simulink model "Lab6CorreguidoMAL"  (R2017b)
settings: Solver=VariableStepAuto  StartTime=0.0  StopTime=10000  RelTol=1e-3
settings Model: Creator=Cx001la  LastModifiedBy=Cx001la

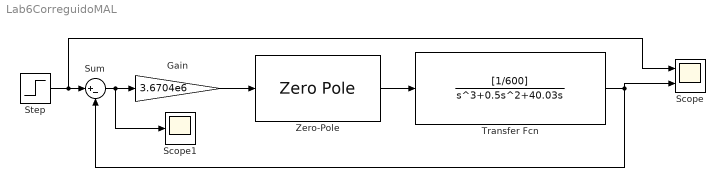
== system Lab6CorreguidoMAL ==
  Gain : Gain  Gain=3.6704e6
  Scope : Scope  NumInputPorts=2
  Scope1 : Scope
  Step : Step  Time=0  SampleTime=0
  Sum : Sum  Inputs=|+-
  Transfer Fcn : TransferFcn  Numerator=[1/600]  Denominator=[1 0.5 40.03 0]
  Zero-Pole : ZeroPole  Zeros=[-2.17 -2.17 -2.17 -2.17 -2.17 ]  Poles=[-18.0788 -18.0788 -18.0788 -18.0788 -18.0788 ]
  wires:
  Step/1 -> Scope/1, Sum/1
  Sum/1 -> Scope1/1, Gain/1
  Gain/1 -> Zero-Pole/1
  Zero-Pole/1 -> Transfer Fcn/1
  Transfer Fcn/1 -> Scope/2, Sum/2
